simulink model "InvDynVarPD"  (R2024b)
settings: Solver=ode15s  StartTime=0.0  StopTime=10  MinStep=0.0000001
InitFcn:
  | addpath('./../Robot Description/Robot Data Package/meshes/visual/')
  | addpath('./../Dynamics and Kinematics/')
  | 
  | % Controller Design
  | Design;
values from neighbouring files (symbols this model uses):
  Kd = 500000    [Design.m]
  Kp = 500000    [Design.m]
  qInitDM = [rand(7, 1); zeros(7, 1)]    [Design.m]
settings Model: Creator=Banaan  LastModifiedBy=Banaan

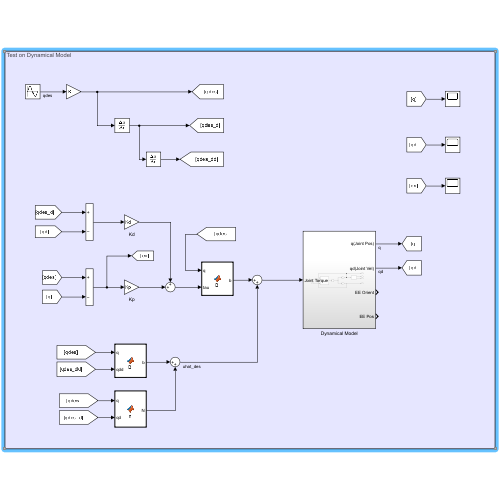
[thumbnail: Simulink's stored preview of the top-level diagram]
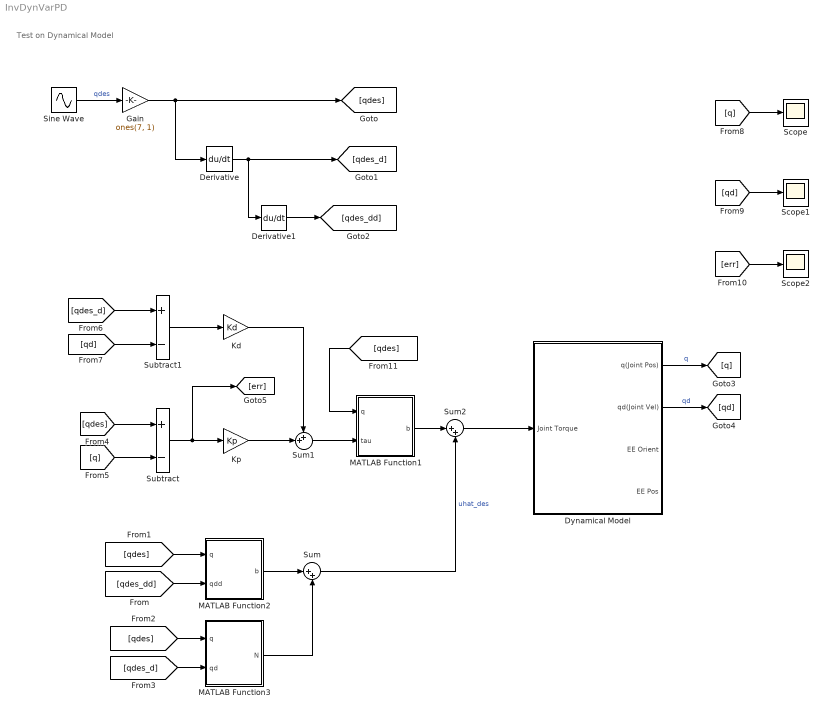
== system InvDynVarPD ==
  note: Test on Dynamical Model
  Derivative : Derivative
  Derivative1 : Derivative
  Dynamical Model : Subsystem
  Gain : Gain  Gain=ones(7, 1)
  Kd : Gain  Gain=Kd
  Kp : Gain  Gain=Kp
  MATLAB Function1 : MATLAB Function  TreatAsAtomicUnit=on
  MATLAB Function2 : MATLAB Function  TreatAsAtomicUnit=on
  MATLAB Function3 : MATLAB Function  TreatAsAtomicUnit=on
  Scope : Scope
  Scope1 : Scope
  Scope2 : Scope
  Sine Wave : Sin  SampleTime=0
  Subtract : Sum  Inputs=+-
  Subtract1 : Sum  Inputs=+-
  Sum : Sum  Inputs=|++
  Sum1 : Sum  Inputs=++|
  Sum2 : Sum  Inputs=|++
  wires:
  Sine Wave/1 -> Gain/1  "qdes"
  Derivative/1 -> Derivative1/1, [qdes_d]
  Derivative1/1 -> [qdes_dd]
  [qdes_dd] -> MATLAB Function2/2(qdd)
  [qdes] -> MATLAB Function2/1(q)
  [qdes_d] -> MATLAB Function3/2(qd)
  [qdes] -> MATLAB Function3/1(q)
  MATLAB Function2/1(b) -> Sum/1
  MATLAB Function3/1(N) -> Sum/2
  Sum1/1 -> MATLAB Function1/2(tau)
  Sum/1 -> Sum2/2  "uhat_des"
  Dynamical Model/1(q(Joint Pos)) -> [q]  "q"
  Dynamical Model/2(qd(Joint Vel)) -> [qd]  "qd"
  Subtract/1 -> [err], Kp/1
  [qdes] -> Subtract/1
  [q] -> Subtract/2
  [qd] -> Subtract1/2
  [qdes_d] -> Subtract1/1
  Subtract1/1 -> Kd/1
  Kd/1 -> Sum1/1
  [q] -> Scope/1
  [qd] -> Scope1/1
  Gain/1 -> [qdes], Derivative/1
  Kp/1 -> Sum1/2
  [err] -> Scope2/1
  Sum2/1 -> Dynamical Model/1(Joint Torque)
  MATLAB Function1/1(b) -> Sum2/1
  [qdes] -> MATLAB Function1/1(q)

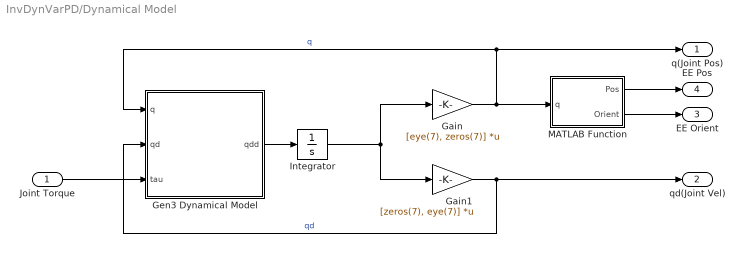
== system InvDynVarPD/Dynamical Model ==
  Joint Torque : Inport
  Gain : Gain  Gain=[eye(7), zeros(7)]  Multiplication=Matrix(K*u)
  Gain1 : Gain  Gain=[zeros(7), eye(7)]  Multiplication=Matrix(K*u)
  Gen3 Dynamical Model : MATLAB Function  TreatAsAtomicUnit=on
  Integrator : Integrator  InitialCondition=qInitDM
  MATLAB Function : MATLAB Function  TreatAsAtomicUnit=on
  q(Joint Pos) : Outport
  qd(Joint Vel) : Outport  Port=2
  EE Orient : Outport  Port=3
  EE Pos : Outport  Port=4
  wires:
  Integrator/1 -> Gain/1, Gain1/1
  Gain/1 -> MATLAB Function/1(q), Gen3 Dynamical Model/1(q), q(Joint Pos)/1  "q"
  Gen3 Dynamical Model/1(qdd) -> Integrator/1
  Gain1/1 -> qd(Joint Vel)/1, Gen3 Dynamical Model/2(qd)  "qd"
  Joint Torque/1 -> Gen3 Dynamical Model/3(tau)
  MATLAB Function/1(Pos) -> EE Pos/1
  MATLAB Function/2(Orient) -> EE Orient/1

== matlab function InvDynVarPD/MATLAB Function2 ==
  data: q input; b output; qdd input
function b = B(q, qdd) %#codegen
    coder.extrinsic('Gen3ODEFun_B');

    tmp = zeros(7, 7);
    tmp = Gen3ODEFun_B(q);

    b = zeros(7, 1);
    b = tmp * qdd;
end

== matlab function InvDynVarPD/Dynamical Model/MATLAB Function ==
  data: q input; Pos output; Orient output
function [Pos, Orient] = FK(q) %#codegen
    coder.extrinsic('Gen3FK');

    tmp = zeros(6, 1);
    tmp = Gen3FK(q);

    Pos    = tmp(1:3, 1);
    Orient = tmp(4:6, 1);      % Order = [Yaw - Pitch - Roll]
end

== matlab function InvDynVarPD/MATLAB Function1 ==
  data: q input; b output; tau input
function b = B(q, tau) %#codegen
    coder.extrinsic('Gen3ODEFun_B');

    tmp = zeros(7, 7);
    tmp = Gen3ODEFun_B(q);

    b = zeros(7, 1);
    b = tmp * tau;
end

== matlab function InvDynVarPD/MATLAB Function3 ==
  data: q input; N output; qd input
function N = n(q, qd) %#codegen
    coder.extrinsic('Gen3ODEFun_C');
    coder.extrinsic('Gen3ODEFun_g');

    N = zeros(7, 1);
    C = zeros(7, 7);
    g = zeros(7, 1);
    
    C = Gen3ODEFun_C(q, qd);
    g = Gen3ODEFun_g(q);
    N = C * qd + g;
end

== matlab function InvDynVarPD/Dynamical Model/Gen3 Dynamical Model ==
  data: q input; qdd output; qd input; tau input
function qdd = fcn(q, qd, tau) %#codegen
    coder.extrinsic('Gen3ODEFun');

    qdd = zeros(14, 1);
    qdd = Gen3ODEFun(0, [q; qd], tau);
end
